simulink model "Exercice2_Simulink"  (R2025b)
settings: Solver=VariableStepAuto  StartTime=0.0  StopTime=4  RelTol=1e-3
libraries: simulink x1
settings Model: Creator=Skander  LastModifiedBy=Skander

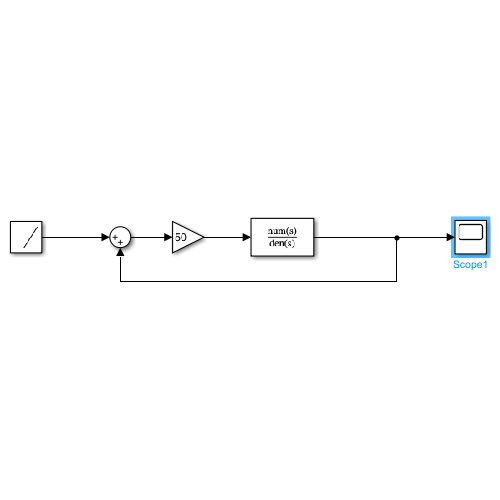
[thumbnail: Simulink's stored preview of the top-level diagram]
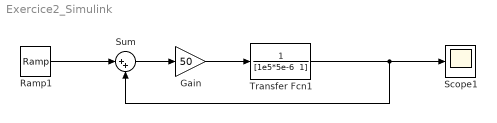
== system Exercice2_Simulink ==
  Gain : Gain  Gain=50
  Ramp1 : simulink/Sources/Ramp  slope=1  start=0  InitialOutput=0
  Scope1 : Scope
      settings: ActiveDisplayYMinimum=-0.067097819109700252  ActiveDisplayYMaximum=0.29681544943833743
  Sum : Sum  Inputs=|++
  Transfer Fcn1 : TransferFcn  Denominator="[1e5*5e-6  1]"
  wires:
  Sum/1 -> Gain/1
  Gain/1 -> Transfer Fcn1/1
  Transfer Fcn1/1 -> Sum/2, Scope1/1
  Ramp1/1 -> Sum/1
